simulink library "SimCoreLib"  (R2016b)
settings: Solver=VariableStepAuto  StartTime=0.0  StopTime=10.0  RelTol=1e-3
undefined symbols (not defined in the file or in its folder): Earth, Env, inertia, m, mass_0, s, Sim, WGS84
undefined symbols (not defined in the file): AC, TrimCondition
libraries: OpenFlightUtilLib x19, SimCoreLib x5, Navigation_Lib x5, aerolib6dofsys x4, aerolibconvert2 x2, SimCore_Lib x1, aerolibutil x1, simulink x1, aerolibtransform2 x1
settings Model: Creator=UAVLAB  LastModifiedBy=rega0051

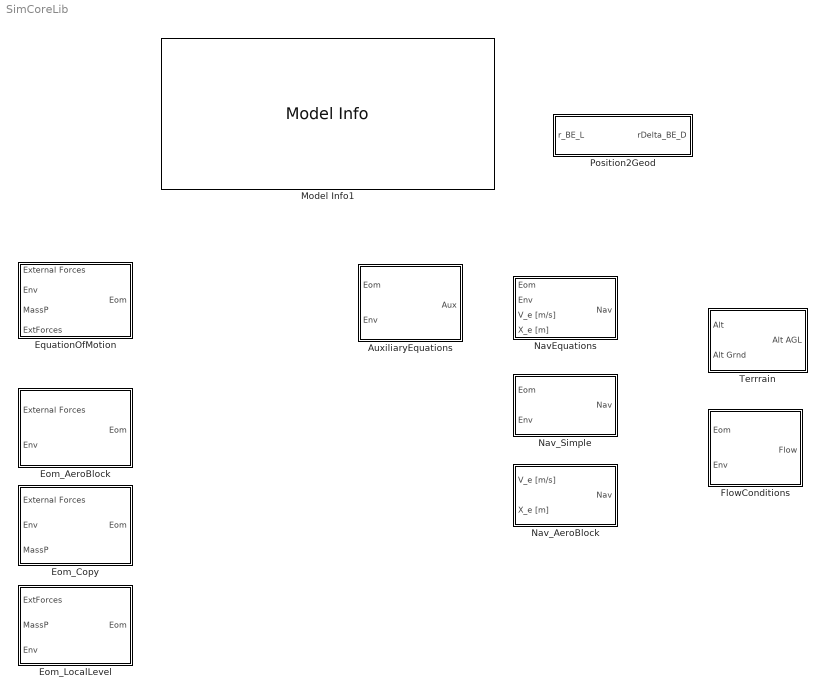
== system SimCoreLib ==
  AuxiliaryEquations : Subsystem
  Eom_AeroBlock : Subsystem  mask(6DoF EoM (Body Axis)){units=Metric (MKS), mtype=Fixed, rep=Euler Angles, xme_0=TrimCondition.InertialIni, Vm_0=TrimCondition.VelocitiesIni, eul_0=TrimCondition.AttitudeIni, pm_0=TrimCondition.RatesIni, mass_0=AC.MassP.mass_kg, mass_e=0.5, mass_f=2.0, inertia=AC.MassP.I_B_kgm2, inertia_e=eye(3), inertia_f=2*eye(3), k_quat=1.0}
      mask prompts: mtype "Mass type:"; rep "Representation:"; xme_0 "Initial position in inertial axes [Xe,Ye,Ze]:"; Vm_0 "Initial velocity in body axes [U,v,w]:"; eul_0 "Initial Euler orientation [roll, pitch, yaw]:"; pm_0 "Initial body rotation rates [p,q,r]:"; mass_0 "Initial mass:"; mass_e "Empty mass:"; mass_f "Full mass:"; inertia_e "Empty inertia matrix:"; inertia_f "Full inertia matrix:"; k_quat "Gain for quaternion normalization:"
      mask help:
      | Integrate the six-degrees-of-freedom equations of motion in body axis.
      |
      | This block has been modified from the original Aerospace Blockset
      | implementation. The inertial position vector (Xe) is no longer computed.
      | The original block did not have a way to add steady state winds to the
      | inertial velocities (Ve) prior to integrating to get Xe. Therefore, this
      | step is performed in the Auxiliary Equations block.
      mask Help: eval('asbhelp(''sixdof_euler_angles'')');
      mask TypeOptions units: Metric (MKS) | English (Velocity in ft/s) | English (Velocity in kts)
      mask TypeOptions mtype: Fixed | Simple Variable | Custom Variable
      mask Callback mtype: aeroicon('aeroblk6dofbody');
      mask TypeOptions rep: Euler Angles | Quaternion
      mask Callback rep: aeroicon('aeroblk6dofbody');
  Eom_Copy : Subsystem  mask{xme_0=TrimCondition.InertialIni, Vm_0=TrimCondition.VelocitiesIni, eul_0=TrimCondition.AttitudeIni, pm_0=TrimCondition.RatesIni, k_quat=1.0}
      mask prompts: xme_0 "Initial position in inertial axes [Xe,Ye,Ze]:"; Vm_0 "Initial velocity in body axes [U,v,w]:"; eul_0 "Initial Euler orientation [roll, pitch, yaw]:"; pm_0 "Initial body rotation rates [p,q,r]:"; k_quat "Gain for quaternion normalization:"
  Eom_LocalLevel : Subsystem
  EquationOfMotion : Subsystem  BlockChoice=Eom_AeroBlock
      settings: TemplateBlock=self  MemberBlocks=Eom_AeroBlock,Eom_Copy,Eom_LocalLevel
  FlowConditions : Subsystem
  Model Info1 : simulink/Model-Wide Utilities/Model Info  Frame=on  DisplayStringWithTags=|  HorizontalTextAlignment=Left  LeftAlignmentValue=0.02  SourceBlockDiagram=SimCoreLib  TagMaxNumber=20
      | MODEL INFORMATION
      | Simulation Core Library (%<ModelName>)
      | 
      | University of Minnesota
      | Aerospace Engineering and Mechanics
      | Copyright 2017 Regents of the University of Minnesota. All rights reserved.
      | 
      | == Update Info ==
      | Last modified by %<LastModifiedBy> on %<LastModificationDate>
  NavEquations : Subsystem  BlockChoice=Nav_Simple
      settings: TemplateBlock=self  MemberBlocks=Nav_AeroBlock,Nav_Simple
  Nav_AeroBlock : Subsystem
  Nav_Simple : Subsystem
  Position2Geod : Subsystem
  Terrrain : Subsystem

== system SimCoreLib/AuxiliaryEquations ==
  Eom : Inport  OutDataTypeStr=Bus: BusEom
  Env : Inport  Port=2  OutDataTypeStr=Bus: BusEnv
  Bus Creator2 : BusCreator  Inputs=2  OutDataTypeStr=Bus: BusAux
      settings: AttributesFormatString=%<OutDataTypeStr>  InheritFromInputs=off
  FlowConditions : SimCoreLib/FlowConditions
  Nav_Simple : SimCoreLib/Nav_Simple
  Aux : Outport
  wires:
  Bus Creator2/1 -> Aux/1  "BusAux"
  Env/1 -> FlowConditions/2, Nav_Simple/2
  Nav_Simple/1 -> Bus Creator2/2
  FlowConditions/1 -> Bus Creator2/1
  Eom/1 -> FlowConditions/1, Nav_Simple/1

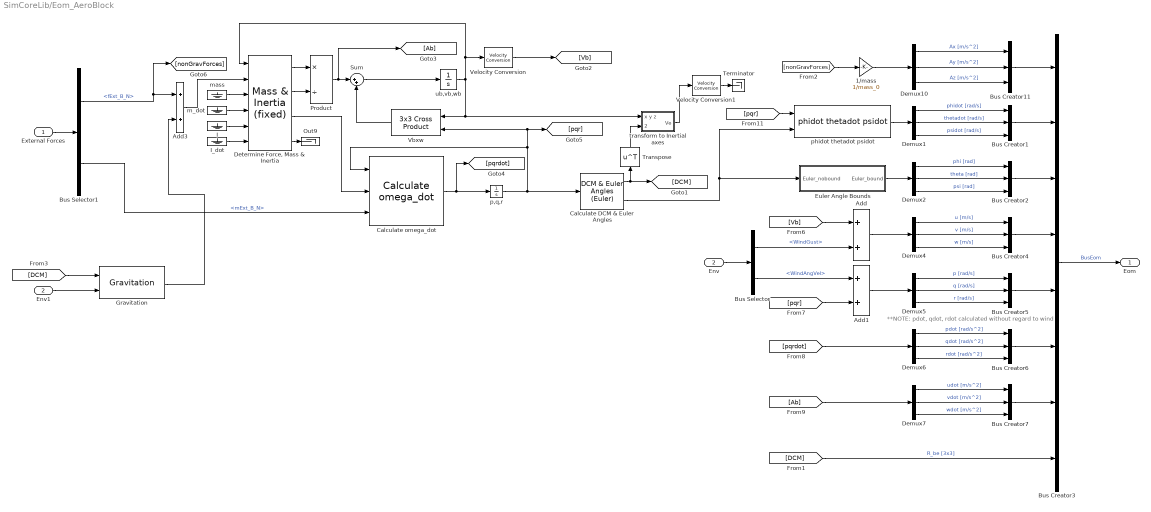
== system SimCoreLib/Eom_AeroBlock ==
  note: **NOTE: pdot, qdot, rdot calculated without regard to wind
  External Forces : Inport
  Env : Inport  Port=2
  1/mass : Gain  Gain=1/mass_0
  Add : Sum
  Add1 : Sum
  Add3 : Sum
  Bus Creator{1..2,4..7,11} (7 alike) : BusCreator  Inputs=3
  Bus Selector : BusSelector  OutputSignals=WindGust,WindAngVel
  Bus Selector1 : BusSelector  OutputSignals=fExt_B_N,mExt_B_N
  Bus Creator3 : BusCreator  Inputs=8  OutDataTypeStr=Bus: BusEom
      settings: AttributesFormatString=%<OutDataTypeStr>  InheritFromInputs=off
  Calculate DCM & Euler Angles : aerolib6dofsys/DCM & Euler Angles (Euler)  SystemSampleTime=-1
  Calculate omega_dot : aerolib6dofsys/Calculate omega_dot  SystemSampleTime=-1
  Demux{1..2,4..7,10} (7 alike) : Demux  Outputs=3
  "Determine Force, Mass & Inertia" : aerolib6dofsys/Mass & Inertia (fixed)  SystemSampleTime=-1
  Env1 : InportShadow  Port=2
  Euler Angle Bounds : Subsystem
  Gravitation : SimCore_Lib/Gravitation
  I : Ground
  I_dot : Ground
  Out9 : Terminator
  Product : Product  Inputs=*/  SaturateOnIntegerOverflow=on  OutDataTypeStr=Inherit: Same as first input
  Sum : Sum  Inputs=|++  SaturateOnIntegerOverflow=on
  Terminator : Terminator
  Transpose : Math  Operator=transpose  SaturateOnIntegerOverflow=on
  Vbxw : aerolibutil/3x3 Cross Product
  Velocity Conversion : aerolibconvert2/Velocity Conversion  IU=m/s  OU=m/s
  Velocity Conversion1 : aerolibconvert2/Velocity Conversion  IU=m/s  OU=m/s
  m_dot : Ground
  mass : Ground
  "p,q,r " : Integrator  InitialCondition=pm_0
  phidot thetadot psidot : aerolib6dofsys/DCM & Euler Angles (Euler)/phidot thetadot psidot
  "transform to Inertial axes " : Subsystem  mask(Vector Transformation){}
      mask Display: disp('L_EB')
  ub,vb,wb : Integrator  InitialCondition=convvel(Vm_0,'m/s','m/s')
  Eom : Outport
  wires:
  [DCM] -> Gravitation/1
  Env1/1 -> Gravitation/2
  Gravitation/1 -> Add3/2
  "Determine Force, Mass & Inertia"/1 -> Product/1
  I_dot/1 -> "Determine Force, Mass & Inertia"/6
  I/1 -> "Determine Force, Mass & Inertia"/5
  Calculate omega_dot/1 -> [pqrdot], "p,q,r "/1
  "Determine Force, Mass & Inertia"/4 -> Out9/1
  m_dot/1 -> "Determine Force, Mass & Inertia"/4
  "Determine Force, Mass & Inertia"/2 -> Product/2
  mass/1 -> "Determine Force, Mass & Inertia"/3
  Transpose/1 -> "transform to Inertial axes "/2(transform coefficients)
  Calculate DCM & Euler Angles/1 -> [DCM], Transpose/1
  Product/1 -> [Ab], Sum/1
  "p,q,r "/1 -> Calculate omega_dot/1, [pqr], Vbxw/2, Calculate DCM & Euler Angles/1
  "transform to Inertial axes "/1(Ve) -> Velocity Conversion1/1
  Sum/1 -> ub,vb,wb/1
  ub,vb,wb/1 -> "Determine Force, Mass & Inertia"/1, Velocity Conversion/1, Vbxw/1, "transform to Inertial axes "/1(x y z)
  Vbxw/1 -> Sum/2
  "Determine Force, Mass & Inertia"/3 -> Calculate omega_dot/2
  Velocity Conversion/1 -> [Vb]
  Velocity Conversion1/1 -> Terminator/1
  Env/1 -> Bus Selector/1
  Bus Selector/1 -> Add/2  "<WindGust>"
  Bus Selector/2 -> Add1/1  "<WindAngVel>"
  [Vb] -> Add/1
  Add/1 -> Demux4/1
  Demux4/3 -> Bus Creator4/3  "w [m/s]"
  Demux4/2 -> Bus Creator4/2  "v [m/s]"
  Demux4/1 -> Bus Creator4/1  "u [m/s]"
  [pqr] -> Add1/2
  Demux5/3 -> Bus Creator5/3  "r [rad/s]"
  Demux5/2 -> Bus Creator5/2  "q [rad/s]"
  Demux5/1 -> Bus Creator5/1  "p [rad/s]"
  Add1/1 -> Demux5/1
  [pqrdot] -> Demux6/1
  Demux6/3 -> Bus Creator6/3  "rdot [rad/s^2]"
  Demux6/2 -> Bus Creator6/2  "qdot [rad/s^2]"
  Demux6/1 -> Bus Creator6/1  "pdot [rad/s^2]"
  [Ab] -> Demux7/1
  Demux7/3 -> Bus Creator7/3  "wdot [m/s^2]"
  Demux7/2 -> Bus Creator7/2  "vdot [m/s^2]"
  Demux7/1 -> Bus Creator7/1  "udot [m/s^2]"
  Demux1/3 -> Bus Creator1/3  "psidot [rad/s]"
  Demux1/2 -> Bus Creator1/2  "thetadot [rad/s]"
  Demux1/1 -> Bus Creator1/1  "phidot [rad/s]"
  phidot thetadot psidot/1 -> Demux1/1
  [pqr] -> phidot thetadot psidot/1
  Calculate DCM & Euler Angles/2 -> Euler Angle Bounds/1(Euler_nobound), phidot thetadot psidot/2
  Demux2/3 -> Bus Creator2/3  "psi [rad]"
  Demux2/2 -> Bus Creator2/2  "theta [rad]"
  Demux2/1 -> Bus Creator2/1  "phi [rad]"
  Euler Angle Bounds/1(Euler_bound) -> Demux2/1
  [nonGravForces] -> 1/mass/1
  1/mass/1 -> Demux10/1
  Demux10/1 -> Bus Creator11/1  "Ax [m/s^2]"
  Demux10/2 -> Bus Creator11/2  "Ay [m/s^2]"
  Demux10/3 -> Bus Creator11/3  "Az [m/s^2]"
  External Forces/1 -> Bus Selector1/1
  Bus Selector1/1 -> [nonGravForces], Add3/1  "<fExt_B_N>"
  Add3/1 -> "Determine Force, Mass & Inertia"/2
  Bus Selector1/2 -> Calculate omega_dot/3  "<mExt_B_N>"
  Bus Creator3/1 -> Eom/1  "BusEom"
  Bus Creator4/1 -> Bus Creator3/4
  Bus Creator5/1 -> Bus Creator3/5
  Bus Creator6/1 -> Bus Creator3/6
  Bus Creator7/1 -> Bus Creator3/7
  Bus Creator1/1 -> Bus Creator3/2
  Bus Creator2/1 -> Bus Creator3/3
  Bus Creator11/1 -> Bus Creator3/1
  [DCM] -> Bus Creator3/8  "R_be [3x3]"

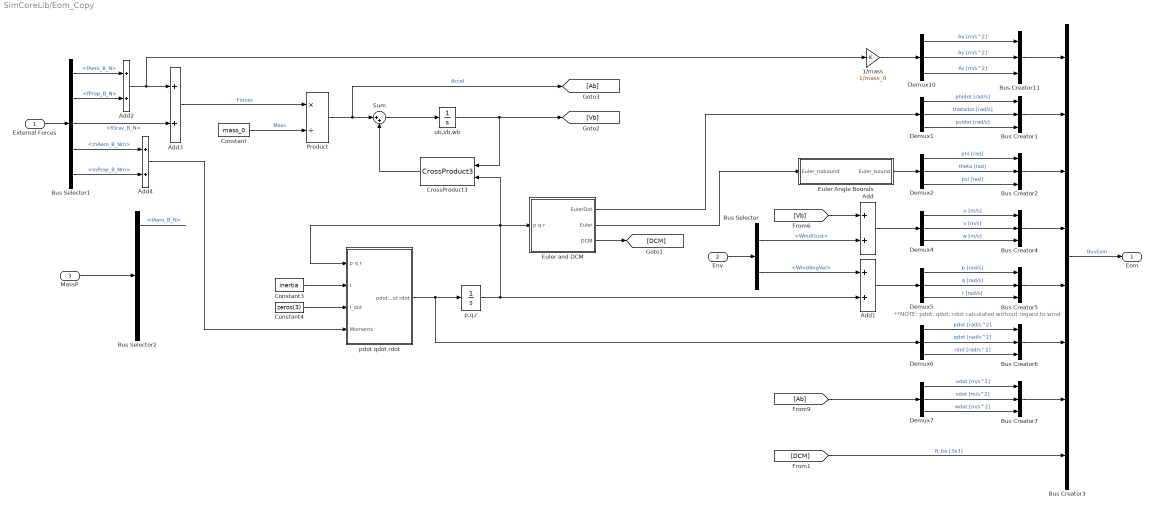
== system SimCoreLib/Eom_Copy ==
  note: **NOTE: pdot, qdot, rdot calculated without regard to wind
  External Forces : Inport
  Env : Inport  Port=2  OutDataTypeStr=Bus: EnvData
  MassP : Inport  Port=3
  1/mass : Gain  Gain=1/mass_0
  Add{,1..4} (5 alike) : Sum
  Bus Creator{1..2,4..7,11} (7 alike) : BusCreator  Inputs=3
  Bus Selector : BusSelector  OutputSignals=WindGust,WindAngVel
  Bus Selector1 : BusSelector  OutputSignals=fAero_B_N,fProp_B_N,fGrav_B_N,mAero_B_Nm,mProp_B_Nm
  Bus Selector2 : BusSelector  OutputSignals=fAero_B_N,fProp_B_N,fGrav_B_N,mAero_B_Nm,mProp_B_Nm
  Bus Creator3 : BusCreator  Inputs=8  OutDataTypeStr=Bus: BusEom
      settings: AttributesFormatString=%<OutDataTypeStr>  InheritFromInputs=off
  Constant : Constant  Value=mass_0  OutDataTypeStr=Inherit: Inherit via back propagation
  Constant3 : Constant  Value=inertia  OutDataTypeStr=Inherit: Inherit via back propagation
  Constant4 : Constant  Value=zeros(3)
  CrossProduct3 : OpenFlightUtilLib/Math/CrossProduct3
  Demux{1..2,4..7,10} (7 alike) : Demux  Outputs=3
  Euler Angle Bounds : Subsystem
  Euler and DCM : Subsystem
  Product : Product  Inputs=*/  SaturateOnIntegerOverflow=on  OutDataTypeStr=Inherit: Same as first input
  Sum : Sum  Inputs=|++  SaturateOnIntegerOverflow=on
  "p,q,r " : Integrator  InitialCondition=pm_0
  pdot qdot rdot : Subsystem
  ub,vb,wb : Integrator  InitialCondition=Vm_0
  Eom : Outport  OutDataTypeStr=Bus: RigidStates
  wires:
  Constant3/1 -> pdot qdot rdot/2(I)
  Constant4/1 -> pdot qdot rdot/3(I_dot)
  ub,vb,wb/1 -> CrossProduct3/1, [Vb]
  Add3/1 -> Product/1  "Forces"
  Constant/1 -> Product/2  "Mass"
  Euler and DCM/3(DCM) -> [DCM]
  Product/1 -> Sum/1, [Ab]  "Accel"
  Sum/1 -> ub,vb,wb/1
  CrossProduct3/1 -> Sum/2
  Env/1 -> Bus Selector/1
  Bus Selector/1 -> Add/2  "<WindGust>"
  Bus Selector/2 -> Add1/1  "<WindAngVel>"
  [Vb] -> Add/1
  Add/1 -> Demux4/1
  Demux4/3 -> Bus Creator4/3  "w [m/s]"
  Demux4/2 -> Bus Creator4/2  "v [m/s]"
  Demux4/1 -> Bus Creator4/1  "u [m/s]"
  "p,q,r "/1 -> pdot qdot rdot/1(p q r), CrossProduct3/2, Euler and DCM/1("p q r "), Add1/2
  Demux5/3 -> Bus Creator5/3  "r [rad/s]"
  Demux5/2 -> Bus Creator5/2  "q [rad/s]"
  Demux5/1 -> Bus Creator5/1  "p [rad/s]"
  Add1/1 -> Demux5/1
  pdot qdot rdot/1(pdot qdot rdot) -> Demux6/1, "p,q,r "/1
  Demux6/3 -> Bus Creator6/3  "rdot [rad/s^2]"
  Demux6/2 -> Bus Creator6/2  "qdot [rad/s^2]"
  Demux6/1 -> Bus Creator6/1  "pdot [rad/s^2]"
  [Ab] -> Demux7/1
  Demux7/3 -> Bus Creator7/3  "wdot [m/s^2]"
  Demux7/2 -> Bus Creator7/2  "vdot [m/s^2]"
  Demux7/1 -> Bus Creator7/1  "udot [m/s^2]"
  Demux1/3 -> Bus Creator1/3  "psidot [rad/s]"
  Demux1/2 -> Bus Creator1/2  "thetadot [rad/s]"
  Demux1/1 -> Bus Creator1/1  "phidot [rad/s]"
  Euler and DCM/1(EulerDot) -> Demux1/1
  Euler and DCM/2(Euler) -> Euler Angle Bounds/1(Euler_nobound)
  Demux2/3 -> Bus Creator2/3  "psi [rad]"
  Demux2/2 -> Bus Creator2/2  "theta [rad]"
  Demux2/1 -> Bus Creator2/1  "phi [rad]"
  Euler Angle Bounds/1(Euler_bound) -> Demux2/1
  Add2/1 -> Add3/1, 1/mass/1
  1/mass/1 -> Demux10/1
  Demux10/1 -> Bus Creator11/1  "Ax [m/s^2]"
  Demux10/2 -> Bus Creator11/2  "Ay [m/s^2]"
  Demux10/3 -> Bus Creator11/3  "Az [m/s^2]"
  External Forces/1 -> Bus Selector1/1
  Bus Selector1/1 -> Add2/1  "<fAero_B_N>"
  Bus Selector1/2 -> Add2/2  "<fProp_B_N>"
  Bus Selector1/3 -> Add3/2  "<fGrav_B_N>"
  Bus Selector1/4 -> Add4/1  "<mAero_B_Nm>"
  Bus Selector1/5 -> Add4/2  "<mProp_B_Nm>"
  Add4/1 -> pdot qdot rdot/4(Moments)
  Bus Creator3/1 -> Eom/1  "BusEom"
  Bus Creator4/1 -> Bus Creator3/4
  Bus Creator5/1 -> Bus Creator3/5
  Bus Creator6/1 -> Bus Creator3/6
  Bus Creator7/1 -> Bus Creator3/7
  Bus Creator1/1 -> Bus Creator3/2
  Bus Creator2/1 -> Bus Creator3/3
  Bus Creator11/1 -> Bus Creator3/1
  [DCM] -> Bus Creator3/8  "R_be [3x3]"
  MassP/1 -> Bus Selector2/1
  Bus Selector2/1 -> ?  "<fAero_B_N>"

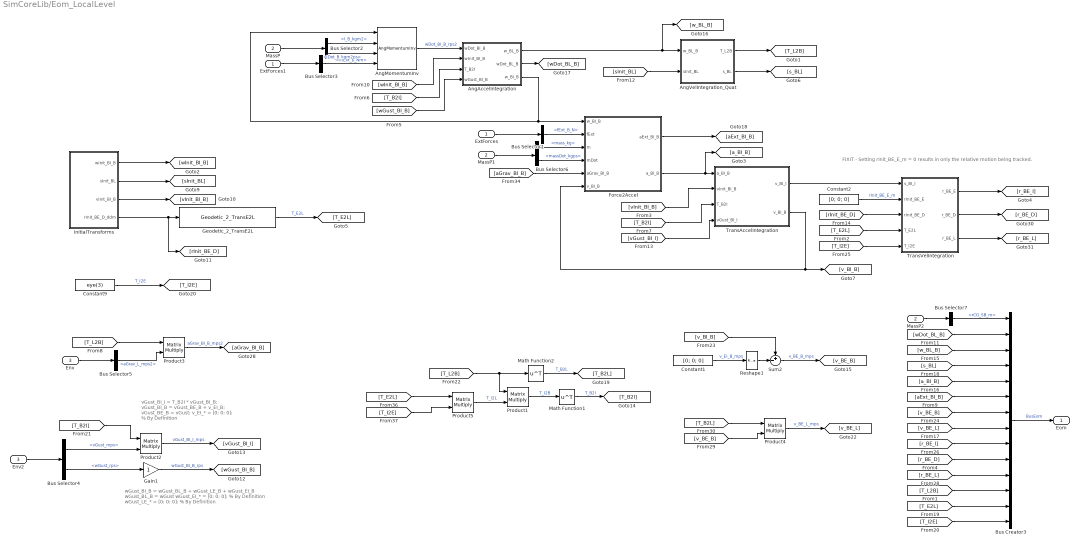
== system SimCoreLib/Eom_LocalLevel ==
  note: wGust_BI_B = wGust_BL_B + wGust_LE_B + wGust_EI_B
      | wGust_BL_B = wGust
      | wGust_EI_* = [0; 0; 0]; % By Definition
      | wGust_LE_* = [0; 0; 0]; % By Definition
  note: vGust_BI_I = T_B2I * vGust_BI_B;
      | vGust_BI_B = vGust_BE_B + v_EI_B;
      | vGust_BE_B = vGust;
      | v_EI_* = [0; 0; 0]; % By Definition
  note: FIXIT - Setting rInit_BE_E_m = 0 results in only the relative motion being tracked.
  ExtForces : Inport
  MassP : Inport  Port=2
  Env : Inport  Port=3  OutDataTypeStr=Bus: BusEnv
  AngAccelIntegration : Subsystem
  AngMomentumInv : OpenFlightUtilLib/Kinematics and Dynamics/AngMomentumInv
  AngVelIntegration_Quat : Subsystem
  Bus Selector1 : BusSelector  OutputSignals=fExt_B_N
  Bus Selector2 : BusSelector  OutputSignals=I_B_kgm2,IDot_B_kgm2ps
  Bus Selector3 : BusSelector  OutputSignals=mExt_B_Nm
  Bus Selector4 : BusSelector  OutputSignals=BusAtmos.vGust_mps,BusAtmos.wGust_rps
  Bus Selector5 : BusSelector  OutputSignals=BusGrav.aGrav_L_mps2
  Bus Selector6 : BusSelector  OutputSignals=mass_kg,massDot_kgps
  Bus Selector7 : BusSelector  OutputSignals=rCG_SB_m
  Bus Creator3 : BusCreator  Inputs=14  OutDataTypeStr=Bus: BusEom
      settings: AttributesFormatString=%<OutDataTypeStr>
  Constant1 : Constant  Value=[0; 0; 0]
      settings: AttributesFormatString=%<Value>
  Constant2 : Constant  Value=[0; 0; 0]
      settings: AttributesFormatString=%<Value>
  Constant9 : Constant  Value=eye(3)
      settings: AttributesFormatString=%<Value>
  Env2 : InportShadow  Port=3  OutDataTypeStr=Bus: BusEnv
  ExtForces1 : InportShadow
  Force2Accel : Subsystem
  Gain1 : Gain
  Geodetic_2_TransE2L : OpenFlightUtilLib/Transformations/Geodetic_2_TransE2L
  InitialTransforms : Subsystem
  MassP1 : InportShadow  Port=2
  MassP2 : InportShadow  Port=2
  Math Function1 : Math  Operator=transpose  SaturateOnIntegerOverflow=on
  Math Function2 : Math  Operator=transpose  SaturateOnIntegerOverflow=on
  Product{1..5} (5 alike) : Product  Inputs=**  Multiplication=Matrix(*)  RndMeth=Zero
  Reshape1 : Reshape  OutputDimensionality=Column vector (2-D)  OutputDimensions=[3,1]
  Sum2 : Sum  Inputs=+-|
  TransAccelIntegration : Subsystem
  TransVelIntegration : Subsystem
  Eom : Outport
  wires:
  Reshape1/1 -> Sum2/2
  Math Function2/1 -> [T_B2L]  "T_B2L"
  [v_BI_B] -> Sum2/1
  Constant1/1 -> Reshape1/1  "v_EI_B_mps"
  Sum2/1 -> [v_BE_B]  "v_BE_B_mps"
  [T_E2L] -> TransVelIntegration/4(T_E2L)
  Constant2/1 -> TransVelIntegration/2(rInit_BE_E)  "rInit_BE_E_m"
  [T_I2E] -> TransVelIntegration/5(T_I2E)
  [r_BE_I] -> Bus Creator3/9
  [v_BE_B] -> Bus Creator3/7
  [vGust_BI_I] -> TransAccelIntegration/4(vGust_BI_I)
  Gain1/1 -> [wGust_BI_B]  "wGust_BI_B_rps"
  Product2/1 -> [vGust_BI_I]  "vGust_BI_I_mps"
  [T_B2I] -> Product2/1
  Bus Selector4/2 -> Gain1/1  "<wGust_rps>"
  Env2/1 -> Bus Selector4/1
  [wGust_BI_B] -> AngAccelIntegration/4(wGust_BI_B)
  Bus Selector7/1 -> Bus Creator3/1  "<rCG_SB_m>"
  MassP2/1 -> Bus Selector7/1
  [T_E2L] -> Product5/1
  [T_I2E] -> Product5/2
  [rInit_BE_D] -> TransVelIntegration/3(rInit_BE_D)
  TransVelIntegration/3(r_BE_L) -> [r_BE_L]
  TransVelIntegration/2(r_BE_D) -> [r_BE_D]
  AngAccelIntegration/2(wDot_BL_B) -> [wDot_BL_B]
  [aGrav_BI_B] -> Force2Accel/5(aGrav_BI_B)
  Bus Selector4/1 -> Product2/2  "<vGust_mps>"
  Product5/1 -> Product1/2  "T_I2L"
  [T_B2L] -> Product4/1
  [v_BE_B] -> Product4/2
  [r_BE_L] -> Bus Creator3/11
  Product4/1 -> [v_BE_L]  "v_BE_L_mps"
  [T_L2B] -> Product1/1, Math Function2/1
  Constant9/1 -> [T_I2E]  "T_I2E"
  Geodetic_2_TransE2L/1 -> [T_E2L]  "T_E2L"
  Force2Accel/1(aExt_BI_B) -> [aExt_BI_B]
  [T_I2E] -> Bus Creator3/14
  [T_E2L] -> Bus Creator3/13
  AngAccelIntegration/1(w_BL_B) -> AngVelIntegration_Quat/1(w_BL_B), [w_BL_B]
  [v_BE_L] -> Bus Creator3/8
  [aExt_BI_B] -> Bus Creator3/6
  [wDot_BL_B] -> Bus Creator3/2
  [w_BL_B] -> Bus Creator3/3
  [r_BE_D] -> Bus Creator3/10
  [a_BI_B] -> Bus Creator3/5
  [s_BL] -> Bus Creator3/4
  MassP1/1 -> Bus Selector6/1
  [wInit_BI_B] -> AngAccelIntegration/2(wInit_BI_B)
  Bus Selector3/1 -> AngMomentumInv/4  "<mExt_B_Nm>"
  Bus Selector2/2 -> AngMomentumInv/3  "<IDot_B_kgm2ps>"
  Bus Selector2/1 -> AngMomentumInv/2  "<I_B_kgm2>"
  AngMomentumInv/1 -> AngAccelIntegration/1(wDot_BI_B)  "wDot_BI_B_rps2"
  [vInit_BI_B] -> TransAccelIntegration/2(vInit_BI_B)
  TransAccelIntegration/2(v_BI_B) -> Force2Accel/6(v_BI_B), [v_BI_B]
  Force2Accel/2(a_BI_B) -> TransAccelIntegration/1(a_BI_B), [a_BI_B]
  AngVelIntegration_Quat/2(s_BL) -> [s_BL]
  [sInit_BL] -> AngVelIntegration_Quat/2(sInit_BL)
  [T_L2B] -> Product3/1
  Bus Selector5/1 -> Product3/2  "<aGrav_L_mps2>"
  Env/1 -> Bus Selector5/1
  ExtForces1/1 -> Bus Selector3/1
  MassP/1 -> Bus Selector2/1
  [T_L2B] -> Bus Creator3/12
  Bus Creator3/1 -> Eom/1  "BusEom"
  Bus Selector1/1 -> Force2Accel/2(fExt)  "<fExt_B_N>"
  ExtForces/1 -> Bus Selector1/1
  AngVelIntegration_Quat/1(T_L2B) -> [T_L2B]
  Product3/1 -> [aGrav_BI_B]  "aGrav_BI_B_mps2"
  Bus Selector6/1 -> Force2Accel/3(m)  "<mass_kg>"
  Bus Selector6/2 -> Force2Accel/4(mDot)  "<massDot_kgps>"
  AngAccelIntegration/3(w_BI_B) -> AngMomentumInv/1, Force2Accel/1(w_BI_B)
  TransAccelIntegration/1(v_BI_I) -> TransVelIntegration/1(v_BI_I)
  TransVelIntegration/1(r_BE_E) -> [r_BE_I]
  [T_B2I] -> AngAccelIntegration/3(T_B2I)
  [T_B2I] -> TransAccelIntegration/3(T_B2I)
  Product1/1 -> Math Function1/1  "T_I2B"
  Math Function1/1 -> [T_B2I]  "T_B2I"
  InitialTransforms/1(wInit_BI_B) -> [wInit_BI_B]
  InitialTransforms/2(sInit_BL) -> [sInit_BL]
  InitialTransforms/3(vInit_BI_B) -> [vInit_BI_B]
  InitialTransforms/4(rInit_BE_D_ddm) -> Geodetic_2_TransE2L/1, [rInit_BE_D]

== system SimCoreLib/EquationOfMotion ==
  External Forces : Inport
  Env : Inport  Port=2
  MassP : Inport  Port=3
  ExtForces : Inport  Port=4
  Eom_AeroBlock : SimCoreLib/Eom_AeroBlock  units=Metric (MKS)  mtype=Fixed  rep=Euler Angles  xme_0=TrimCondition.InertialIni  Vm_0=TrimCondition.VelocitiesIni  eul_0=TrimCondition.AttitudeIni  pm_0=TrimCondition.RatesIni  mass_0=AC.MassP.mass_kg  mass_e=0.5  mass_f=2.0  inertia=AC.MassP.I_B_kgm2  inertia_e=eye(3)  inertia_f=2*eye(3)  k_quat=1.0
  term3 : Terminator
  term4 : Terminator
  Eom : Outport
  wires:
  External Forces/1 -> Eom_AeroBlock/1
  Env/1 -> Eom_AeroBlock/2
  Eom_AeroBlock/1 -> Eom/1
  MassP/1 -> term3/1
  ExtForces/1 -> term4/1

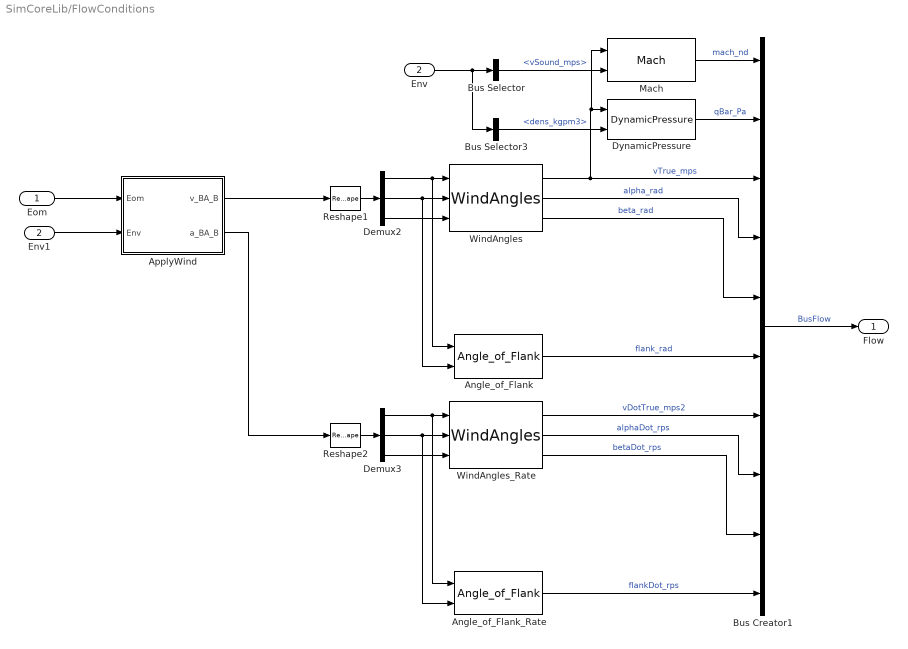
== system SimCoreLib/FlowConditions ==
  Eom : Inport
  Env : Inport  Port=2
  Angle_of_Flank : OpenFlightUtilLib/Air Data/Angle_of_Flank
  Angle_of_Flank_Rate : OpenFlightUtilLib/Air Data/Angle_of_Flank
  ApplyWind : Subsystem
  Bus Creator1 : BusCreator  Inputs=10  OutDataTypeStr=Bus: BusFlow
      settings: InheritFromInputs=off
  Bus Selector : BusSelector  OutputSignals=BusAtmos.vSound_mps
  Bus Selector3 : BusSelector  OutputSignals=BusAtmos.dens_kgpm3
  Demux2 : Demux  Outputs=3
  Demux3 : Demux  Outputs=3
  DynamicPressure : OpenFlightUtilLib/Air Data/DynamicPressure
  Env1 : InportShadow  Port=2
  Mach : OpenFlightUtilLib/Air Data/Mach
  Reshape1 : Reshape  OutputDimensions=[3,1]
  Reshape2 : Reshape  OutputDimensions=[3,1]
  WindAngles : OpenFlightUtilLib/Air Data/WindAngles
  WindAngles_Rate : OpenFlightUtilLib/Air Data/WindAngles
  Flow : Outport
  wires:
  Reshape2/1 -> Demux3/1
  Reshape1/1 -> Demux2/1
  ApplyWind/2(a_BA_B) -> Reshape2/1
  Env1/1 -> ApplyWind/2(Env)
  Eom/1 -> ApplyWind/1(Eom)
  WindAngles_Rate/2 -> Bus Creator1/8  "alphaDot_rps"
  Demux3/2 -> Angle_of_Flank_Rate/2, WindAngles_Rate/2
  WindAngles_Rate/1 -> Bus Creator1/7  "vDotTrue_mps2"
  Demux3/3 -> WindAngles_Rate/3
  Demux3/1 -> Angle_of_Flank_Rate/1, WindAngles_Rate/1
  WindAngles_Rate/3 -> Bus Creator1/9  "betaDot_rps"
  WindAngles/3 -> Bus Creator1/5  "beta_rad"
  Angle_of_Flank/1 -> Bus Creator1/6  "flank_rad"
  Angle_of_Flank_Rate/1 -> Bus Creator1/10  "flankDot_rps"
  Bus Creator1/1 -> Flow/1  "BusFlow"
  WindAngles/2 -> Bus Creator1/4  "alpha_rad"
  Demux2/2 -> Angle_of_Flank/2, WindAngles/2
  Demux2/1 -> Angle_of_Flank/1, WindAngles/1
  WindAngles/1 -> Mach/1, DynamicPressure/1, Bus Creator1/3  "vTrue_mps"
  Demux2/3 -> WindAngles/3
  DynamicPressure/1 -> Bus Creator1/2  "qBar_Pa"
  Bus Selector3/1 -> DynamicPressure/2  "<dens_kgpm3>"
  Env/1 -> Bus Selector3/1, Bus Selector/1
  Bus Selector/1 -> Mach/2  "<vSound_mps>"
  Mach/1 -> Bus Creator1/1  "mach_nd"
  ApplyWind/1(v_BA_B) -> Reshape1/1

== system SimCoreLib/NavEquations ==
  Eom : Inport
  Env : Inport  Port=2
  V_e [m/s] : Inport  Port=3
  X_e [m] : Inport  Port=4
  Nav_Simple : SimCoreLib/Nav_Simple
  term3 : Terminator
  term4 : Terminator
  Nav : Outport
  wires:
  Eom/1 -> Nav_Simple/1
  Env/1 -> Nav_Simple/2
  Nav_Simple/1 -> Nav/1
  V_e [m/s]/1 -> term3/1
  X_e [m]/1 -> term4/1

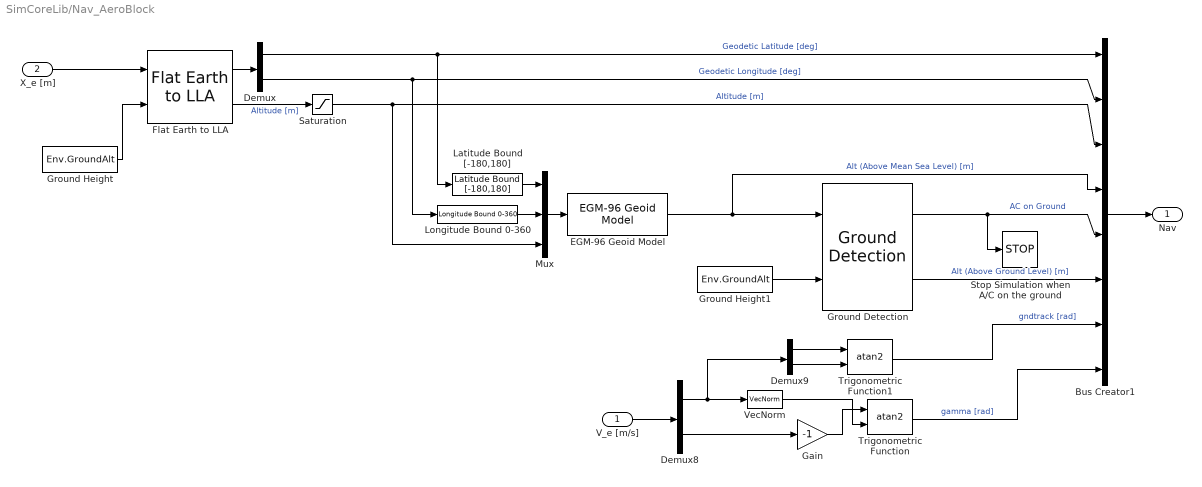
== system SimCoreLib/Nav_AeroBlock ==
  V_e [m/s] : Inport
  X_e [m] : Inport  Port=2
  Bus Creator1 : BusCreator  Inputs=8  OutDataTypeStr=Bus: Nav
      settings: InheritFromInputs=off
  Demux : Demux  Outputs=2
  Demux8 : Demux  Outputs=[2 1]
  Demux9 : Demux  Outputs=2
  EGM-96 Geoid Model : Navigation_Lib/Navigation/EGM-96 Geoid Model
  Flat Earth to LLA : aerolibtransform2/Flat Earth to LLA  units=Metric (MKS)  ptype=Earth (WGS84)  F=1/298.257223563  R=6378137  LL0=TrimCondition.LLIni  psi=0
  Gain : Gain  Gain=-1
  Ground Detection : Navigation_Lib/Navigation/Ground Detection
  Ground Height : Constant  Value=Env.GroundAlt
  Ground Height1 : Constant  Value=Env.GroundAlt
  Latitude Bound [-180,180] : Navigation_Lib/Navigation/Latitude Bound [-180,180]
  Longitude Bound 0-360 : Navigation_Lib/Navigation/Longitude Bound 0-360
  Mux : Mux  Inputs=3
  Saturation : Saturate  UpperLimit=Inf  LowerLimit=0
  Stop Simulation when A/C on the ground : Stop
  Trigonometric Function : Trigonometry  Operator=atan2
  Trigonometric Function1 : Trigonometry  Operator=atan2
  VecNorm : Navigation_Lib/Navigation/VecNorm
  Nav : Outport  OutDataTypeStr=Bus: Nav
  wires:
  Flat Earth to LLA/1 -> Demux/1
  Flat Earth to LLA/2 -> Saturation/1  "Altitude [m]"
  Demux/1 -> Bus Creator1/1, Latitude Bound [-180,180]/1  "Geodetic Latitude [deg]"
  Demux/2 -> Bus Creator1/2, Longitude Bound 0-360/1  "Geodetic Longitude [deg]"
  X_e [m]/1 -> Flat Earth to LLA/1
  Ground Height/1 -> Flat Earth to LLA/2
  Bus Creator1/1 -> Nav/1
  EGM-96 Geoid Model/1 -> Ground Detection/1, Bus Creator1/4  "Alt (Above Mean Sea Level) [m]"
  Ground Height1/1 -> Ground Detection/2
  Ground Detection/1 -> Stop Simulation when A/C on the ground/1, Bus Creator1/5  "AC on Ground"
  Saturation/1 -> Bus Creator1/3, Mux/3  "Altitude [m]"
  Mux/1 -> EGM-96 Geoid Model/1
  Ground Detection/2 -> Bus Creator1/6  "Alt (Above Ground Level) [m]"
  V_e [m/s]/1 -> Demux8/1
  Demux8/2 -> Gain/1
  VecNorm/1 -> Trigonometric Function/2
  Trigonometric Function/1 -> Bus Creator1/8  "gamma [rad]"
  Demux9/2 -> Trigonometric Function1/2
  Trigonometric Function1/1 -> Bus Creator1/7  "gndtrack [rad]"
  Demux8/1 -> VecNorm/1, Demux9/1
  Demux9/1 -> Trigonometric Function1/1
  Longitude Bound 0-360/1 -> Mux/2
  Latitude Bound [-180,180]/1 -> Mux/1
  Gain/1 -> Trigonometric Function/1

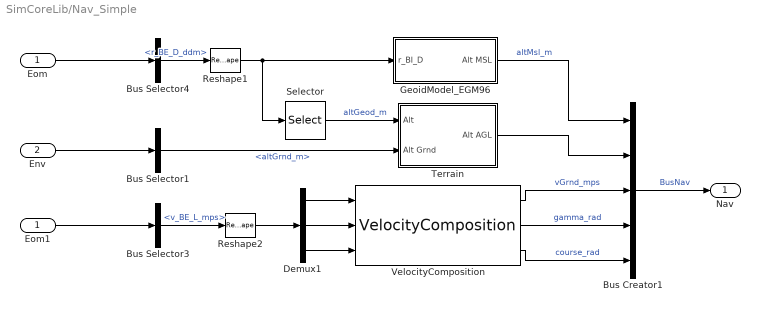
== system SimCoreLib/Nav_Simple ==
  Eom : Inport
  Env : Inport  Port=2
  Bus Creator1 : BusCreator  Inputs=5  OutDataTypeStr=Bus: BusNav
      settings: AttributesFormatString=%<OutDataTypeStr>  InheritFromInputs=off
  Bus Selector1 : BusSelector  OutputSignals=BusTerr.altGrnd_m
  Bus Selector3 : BusSelector  OutputSignals=v_BE_L_mps
  Bus Selector4 : BusSelector  OutputSignals=r_BE_D_ddm
  Demux1 : Demux  Outputs=3
  Eom1 : InportShadow
  GeoidModel_EGM96 : Subsystem  mask(EGM-96 geoid undulation model){}
      mask help: Computes the MSL (mean sea level) altitude as a function of position.
      mask init:
      | load('egm96');
      mask Help:
      | The block computes the mean-sea-level altitude relative to the WGS-84 geoid.
      | <P><B>Inputs:</B>
      | <LI>Position = the 3x1 vector of aircraft location [Latitude Longitude Altitude], in [rad rad m]</LI>
      | </P>
      | <P><B>Output:</B>
      | <LI>MSLAlt = the mean-sea-level altitude, in m</LI>
      | </P>
  Reshape1 : Reshape  OutputDimensions=[3,1]
  Reshape2 : Reshape  OutputDimensions=[3,1]
  Selector : Selector  InputPortWidth=3  IndexOptions=Index vector (dialog)  Indices=3  OutputSizes=1
  Terrain : Subsystem
  VelocityComposition : OpenFlightUtilLib/Transformations/VelocityComposition
  Nav : Outport
  wires:
  Reshape2/1 -> Demux1/1
  Reshape1/1 -> Selector/1, GeoidModel_EGM96/1(r_BI_D)
  Bus Selector4/1 -> Reshape1/1  "<r_BE_D_ddm>"
  Bus Selector3/1 -> Reshape2/1  "<v_BE_L_mps>"
  Eom1/1 -> Bus Selector3/1
  Bus Creator1/1 -> Nav/1  "BusNav"
  GeoidModel_EGM96/1(Alt MSL) -> Bus Creator1/1  "altMsl_m"
  Selector/1 -> Terrain/1(Alt)  "altGeod_m"
  Demux1/1 -> VelocityComposition/1
  Demux1/2 -> VelocityComposition/2
  Demux1/3 -> VelocityComposition/3
  VelocityComposition/1 -> Bus Creator1/3  "vGrnd_mps"
  VelocityComposition/2 -> Bus Creator1/4  "gamma_rad"
  VelocityComposition/3 -> Bus Creator1/5  "course_rad"
  Eom/1 -> Bus Selector4/1
  Terrain/1(Alt AGL) -> Bus Creator1/2
  Bus Selector1/1 -> Terrain/2(Alt Grnd)  "<altGrnd_m>"
  Env/1 -> Bus Selector1/1

== system SimCoreLib/Position2Geod ==
  r_BE_L : Inport
  Constant1 : Constant  Value=Env.Earth.radiusEquator_m
      settings: AttributesFormatString=%<Value>
  Constant2 : Constant  Value=Env.Earth.radiusPolar_m
      settings: AttributesFormatString=%<Value>
  Demux1 : Demux  Outputs=3
  Gain : Gain  Gain=180/pi
      settings: AttributesFormatString=%<Gain>
  Gain1 : Gain  Gain=-1
      settings: AttributesFormatString=%<Gain>
  Gain2 : Gain  Gain=180/pi
      settings: AttributesFormatString=%<Gain>
  Mux : Mux  Inputs=3
  Product : Product  Inputs=*/
  Product1 : Product  Inputs=*/
  rDelta_BE_D : Outport
  wires:
  Gain1/1 -> Mux/3
  Mux/1 -> rDelta_BE_D/1  "rDelta_BE_D_ddm"
  Demux1/3 -> Gain1/1
  Demux1/1 -> Product/1
  Constant2/1 -> Product/2
  r_BE_L/1 -> Demux1/1
  Gain2/1 -> Mux/1
  Product/1 -> Gain2/1
  Constant1/1 -> Product1/2
  Demux1/2 -> Product1/1
  Product1/1 -> Gain/1
  Gain/1 -> Mux/2

== system SimCoreLib/Terrrain ==
  Alt : Inport
  Alt Grnd : Inport  Port=2
  Sum : Sum  Inputs=|+-  SaturateOnIntegerOverflow=on  InputSameDT=on  OutDataTypeStr=Inherit: Same as first input
  Alt AGL : Outport
  wires:
  Alt/1 -> Sum/1
  Sum/1 -> Alt AGL/1  "altAgl_m"
  Alt Grnd/1 -> Sum/2

== system SimCoreLib/Eom_AeroBlock/Euler Angle Bounds ==
  Euler_nobound : Inport
  2pi Bound : Subsystem
  Demux : Demux  Outputs=3
  Mux : Mux  Inputs=3
  pi Bound : Subsystem
  pi/2 Bound : Subsystem
  Euler_bound : Outport
  wires:
  pi Bound/1(Out) -> Mux/2
  pi/2 Bound/1(Out) -> Mux/1
  Mux/1 -> Euler_bound/1
  Euler_nobound/1 -> Demux/1
  Demux/1 -> pi/2 Bound/1(In)
  Demux/2 -> pi Bound/1(In)
  Demux/3 -> 2pi Bound/1(In)
  2pi Bound/1(Out) -> Mux/3

== system SimCoreLib/Eom_AeroBlock/transform to Inertial axes  ==
  x y z : Inport
  transform coefficients : Inport  Port=2
  Product : Product  Multiplication=Matrix(*)  SaturateOnIntegerOverflow=on  InputSameDT=on  OutDataTypeStr=Inherit: Same as first input
  Reshape1 : Reshape  OutputDimensionality=Column vector (2-D)
  Reshape2 : Reshape
  Ve : Outport
  wires:
  Reshape2/1 -> Ve/1
  Reshape1/1 -> Product/2
  x y z/1 -> Reshape1/1
  transform coefficients/1 -> Product/1
  Product/1 -> Reshape2/1

== system SimCoreLib/Eom_Copy/Euler Angle Bounds ==
  Euler_nobound : Inport
  2pi Bound : Subsystem
  Demux : Demux  Outputs=3
  Mux : Mux  Inputs=3
  pi Bound : Subsystem
  pi/2 Bound : Subsystem
  Euler_bound : Outport
  wires:
  2pi Bound/1(Out) -> Mux/3
  Demux/3 -> 2pi Bound/1(In)
  Demux/2 -> pi Bound/1(In)
  Demux/1 -> pi/2 Bound/1(In)
  Euler_nobound/1 -> Demux/1
  Mux/1 -> Euler_bound/1
  pi/2 Bound/1(Out) -> Mux/1
  pi Bound/1(Out) -> Mux/2

== system SimCoreLib/Eom_Copy/Euler and DCM ==
  "p q r " : Inport
  DCM_321 : OpenFlightUtilLib/Transformations/DCM_321
  Demux3 : Demux  Outputs=3
  phi theta psi : Integrator  InitialCondition=eul_0
  phidot thetadot psidot : Subsystem
  EulerDot : Outport
  Euler : Outport  Port=2
  DCM : Outport  Port=3
  wires:
  Demux3/1 -> DCM_321/1
  Demux3/2 -> DCM_321/2
  Demux3/3 -> DCM_321/3
  DCM_321/1 -> DCM/1
  "p q r "/1 -> phidot thetadot psidot/2(p q r)
  phidot thetadot psidot/1(phidt thetadt psidt) -> phi theta psi/1, EulerDot/1
  phi theta psi/1 -> Euler/1, Demux3/1, phidot thetadot psidot/1(phi theta psi)

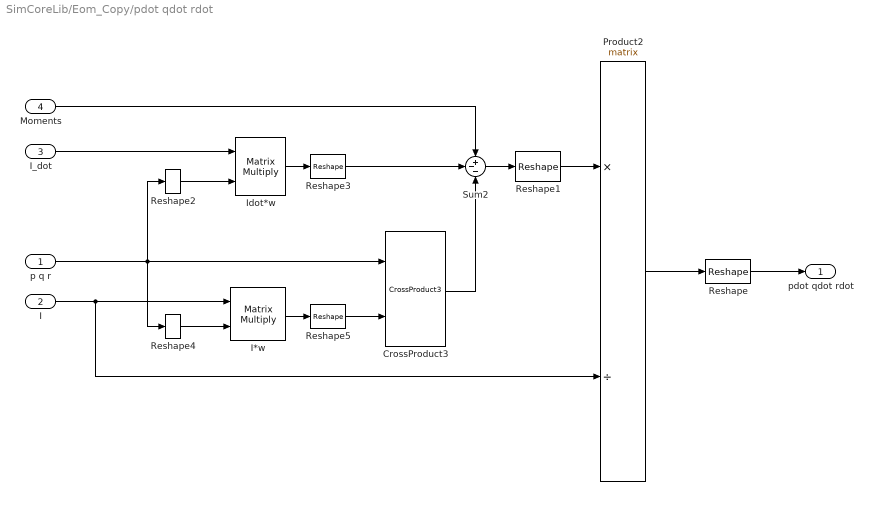
== system SimCoreLib/Eom_Copy/pdot qdot rdot ==
  p q r : Inport
  I : Inport  Port=2
  I_dot : Inport  Port=3
  Moments : Inport  Port=4
  CrossProduct3 : OpenFlightUtilLib/Math/CrossProduct3
  I*w : Product  Multiplication=Matrix(*)  SaturateOnIntegerOverflow=on  InputSameDT=on  OutDataTypeStr=Inherit: Same as first input
  Idot*w : Product  Multiplication=Matrix(*)  SaturateOnIntegerOverflow=on  InputSameDT=on  OutDataTypeStr=Inherit: Same as first input
  Product2 : Product  Inputs=*/  Multiplication=Matrix(*)  SaturateOnIntegerOverflow=on  OutDataTypeStr=Inherit: Same as first input
  Reshape : Reshape
  Reshape1 : Reshape  OutputDimensionality=Row vector (2-D)
  Reshape2 : Reshape  OutputDimensionality=Column vector (2-D)
  Reshape3 : Reshape
  Reshape4 : Reshape  OutputDimensionality=Column vector (2-D)
  Reshape5 : Reshape
  Sum2 : Sum  Inputs=+--  SaturateOnIntegerOverflow=on
  pdot qdot rdot : Outport
  wires:
  I*w/1 -> Reshape5/1
  I/1 -> I*w/1, Product2/2
  Reshape4/1 -> I*w/2
  I_dot/1 -> Idot*w/1
  Idot*w/1 -> Reshape3/1
  Reshape2/1 -> Idot*w/2
  Reshape/1 -> pdot qdot rdot/1
  p q r/1 -> CrossProduct3/1, Reshape4/1, Reshape2/1
  Product2/1 -> Reshape/1
  Sum2/1 -> Reshape1/1
  Moments/1 -> Sum2/1
  Reshape3/1 -> Sum2/2
  CrossProduct3/1 -> Sum2/3
  Reshape5/1 -> CrossProduct3/2
  Reshape1/1 -> Product2/1

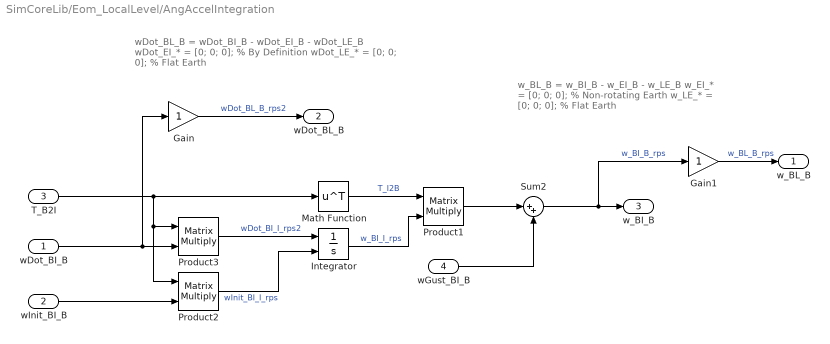
== system SimCoreLib/Eom_LocalLevel/AngAccelIntegration ==
  note: w_BL_B = w_BI_B - w_EI_B - w_LE_B
      | w_EI_* = [0; 0; 0]; % Non-rotating Earth
      | w_LE_* = [0; 0; 0]; % Flat Earth
  note: wDot_BL_B = wDot_BI_B - wDot_EI_B - wDot_LE_B
      | wDot_EI_* = [0; 0; 0]; % By Definition
      | wDot_LE_* = [0; 0; 0]; % Flat Earth
  wDot_BI_B : Inport
  wInit_BI_B : Inport  Port=2
  T_B2I : Inport  Port=3
  wGust_BI_B : Inport  Port=4
  Gain : Gain
  Gain1 : Gain
  Integrator : Integrator  InitialConditionSource=external  ContinuousStateAttributes='wState_BI_I_rps'
      settings: AttributesFormatString=State: %<ContinuousStateAttributes>
  Math Function : Math  Operator=transpose  SaturateOnIntegerOverflow=on
  Product1 : Product  Inputs=**  Multiplication=Matrix(*)  RndMeth=Zero
  Product2 : Product  Inputs=**  Multiplication=Matrix(*)  RndMeth=Zero
  Product3 : Product  Inputs=**  Multiplication=Matrix(*)  RndMeth=Zero
  Sum2 : Sum  Inputs=|++  SaturateOnIntegerOverflow=on
  w_BL_B : Outport
  wDot_BL_B : Outport  Port=2
  w_BI_B : Outport  Port=3
  wires:
  Product1/1 -> Sum2/1
  wGust_BI_B/1 -> Sum2/2
  Gain/1 -> wDot_BL_B/1  "wDot_BL_B_rps2"
  Gain1/1 -> w_BL_B/1  "w_BL_B_rps"
  wDot_BI_B/1 -> Product3/2, Gain/1
  Product2/1 -> Integrator/2  "wInit_BI_I_rps"
  wInit_BI_B/1 -> Product2/2
  Integrator/1 -> Product1/2  "w_BI_I_rps"
  T_B2I/1 -> Math Function/1, Product3/1, Product2/1
  Product3/1 -> Integrator/1  "wDot_BI_I_rps2"
  Math Function/1 -> Product1/1  "T_I2B"
  Sum2/1 -> w_BI_B/1, Gain1/1  "w_BI_B_rps"

== system SimCoreLib/Eom_LocalLevel/AngVelIntegration_Quat ==
  w_BL_B : Inport
  sInit_BL : Inport  Port=2
  Euler2Quat : OpenFlightUtilLib/Transformations/Euler2Quat
  NormL2 : OpenFlightUtilLib/Math/NormL2
  Product2 : Product  Inputs=*/  RndMeth=Zero
  Quat2DCM321 : OpenFlightUtilLib/Transformations/Quat2DCM
  Quat2Euler : OpenFlightUtilLib/Transformations/Quat2Euler
  QuatDeriv : OpenFlightUtilLib/Transformations/QuatDeriv
  QuatInt : OpenFlightUtilLib/Transformations/QuatInt
  T_L2B : Outport
  s_BL : Outport  Port=2
  wires:
  sInit_BL/1 -> Euler2Quat/1
  Quat2Euler/1 -> s_BL/1  "s_BL_rad"
  Quat2DCM321/1 -> T_L2B/1  "T_L2B"
  NormL2/1 -> Product2/2
  QuatDeriv/1 -> QuatInt/1  "quatDot_BL_nd"
  QuatInt/1 -> Product2/1, NormL2/1
  Product2/1 -> Quat2Euler/1, Quat2DCM321/1, QuatDeriv/1  "quat_BL_nd"
  Euler2Quat/1 -> QuatInt/2  "quatInit_BL_nd"
  w_BL_B/1 -> QuatDeriv/2

== system SimCoreLib/Eom_LocalLevel/Force2Accel ==
  w_BI_B : Inport
  fExt : Inport  Port=2
  m : Inport  Port=3
  mDot : Inport  Port=4
  aGrav_BI_B : Inport  Port=5
  v_BI_B : Inport  Port=6
  Sum2 : Sum  Inputs=|++  SaturateOnIntegerOverflow=on
  TransMomentumInv : OpenFlightUtilLib/Kinematics and Dynamics/TransMomentumInv
  aExt_BI_B : Outport
  a_BI_B : Outport  Port=2
  wires:
  fExt/1 -> TransMomentumInv/3
  v_BI_B/1 -> TransMomentumInv/1
  TransMomentumInv/1 -> Sum2/1, aExt_BI_B/1  "aExt_BI_B_mps2"
  w_BI_B/1 -> TransMomentumInv/5
  mDot/1 -> TransMomentumInv/4
  m/1 -> TransMomentumInv/2
  aGrav_BI_B/1 -> Sum2/2
  Sum2/1 -> a_BI_B/1  "a_BI_B_mps2"

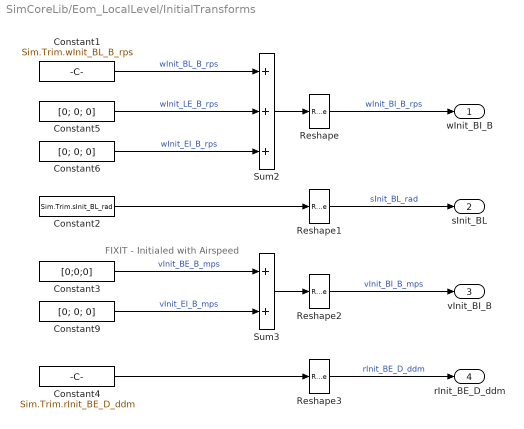
== system SimCoreLib/Eom_LocalLevel/InitialTransforms ==
  note: FIXIT - Initialed with Airspeed
  Constant1 : Constant  Value=Sim.Trim.wInit_BL_B_rps
      settings: AttributesFormatString=%<Value>
  Constant2 : Constant  Value=Sim.Trim.sInit_BL_rad
      settings: AttributesFormatString=%<Value>
  Constant3 : Constant  Value=[0;0;0]
      settings: AttributesFormatString=%<Value>
  Constant4 : Constant  Value=Sim.Trim.rInit_BE_D_ddm
      settings: AttributesFormatString=%<Value>
  Constant5 : Constant  Value=[0; 0; 0]
      settings: AttributesFormatString=%<Value>
  Constant6 : Constant  Value=[0; 0; 0]
      settings: AttributesFormatString=%<Value>
  Constant9 : Constant  Value=[0; 0; 0]
      settings: AttributesFormatString=%<Value>
  Reshape{,1..3} (4 alike) : Reshape  OutputDimensionality=Column vector (2-D)  OutputDimensions=[3,1]
  Sum2 : Sum  Inputs=+++  SaturateOnIntegerOverflow=on
  Sum3 : Sum  SaturateOnIntegerOverflow=on
  wInit_BI_B : Outport
  sInit_BL : Outport  Port=2
  vInit_BI_B : Outport  Port=3
  rInit_BE_D_ddm : Outport  Port=4
  wires:
  Reshape3/1 -> rInit_BE_D_ddm/1  "rInit_BE_D_ddm"
  Reshape2/1 -> vInit_BI_B/1  "vInit_BI_B_mps"
  Reshape1/1 -> sInit_BL/1  "sInit_BL_rad"
  Sum2/1 -> Reshape/1
  Sum3/1 -> Reshape2/1
  Constant9/1 -> Sum3/2  "vInit_EI_B_mps"
  Constant6/1 -> Sum2/3  "wInit_EI_B_rps"
  Constant5/1 -> Sum2/2  "wInit_LE_B_rps"
  Reshape/1 -> wInit_BI_B/1  "wInit_BI_B_rps"
  Constant4/1 -> Reshape3/1
  Constant3/1 -> Sum3/1  "vInit_BE_B_mps"
  Constant2/1 -> Reshape1/1
  Constant1/1 -> Sum2/1  "wInit_BL_B_rps"

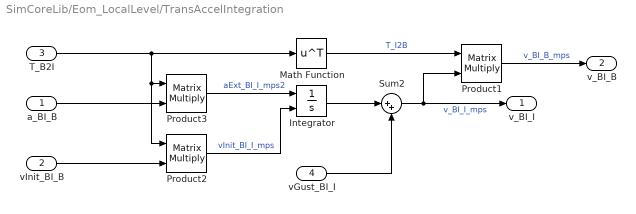
== system SimCoreLib/Eom_LocalLevel/TransAccelIntegration ==
  a_BI_B : Inport
  vInit_BI_B : Inport  Port=2
  T_B2I : Inport  Port=3
  vGust_BI_I : Inport  Port=4
  Integrator : Integrator  InitialConditionSource=external  ContinuousStateAttributes='vState_BI_I_mps'
      settings: AttributesFormatString=State: %<ContinuousStateAttributes>
  Math Function : Math  Operator=transpose  SaturateOnIntegerOverflow=on
  Product1 : Product  Inputs=**  Multiplication=Matrix(*)  RndMeth=Zero
  Product2 : Product  Inputs=**  Multiplication=Matrix(*)  RndMeth=Zero
  Product3 : Product  Inputs=**  Multiplication=Matrix(*)  RndMeth=Zero
  Sum2 : Sum  Inputs=|++  SaturateOnIntegerOverflow=on
  v_BI_I : Outport
  v_BI_B : Outport  Port=2
  wires:
  Integrator/1 -> Sum2/1
  vGust_BI_I/1 -> Sum2/2
  Sum2/1 -> v_BI_I/1, Product1/2  "v_BI_I_mps"
  vInit_BI_B/1 -> Product2/2
  a_BI_B/1 -> Product3/2
  T_B2I/1 -> Product3/1, Product2/1, Math Function/1
  Math Function/1 -> Product1/1  "T_I2B"
  Product1/1 -> v_BI_B/1  "v_BI_B_mps"
  Product3/1 -> Integrator/1  "aExt_BI_I_mps2"
  Product2/1 -> Integrator/2  "vInit_BI_I_mps"

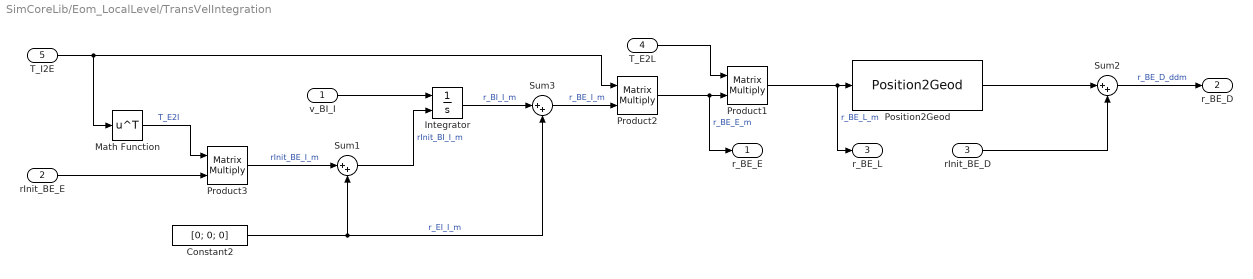
== system SimCoreLib/Eom_LocalLevel/TransVelIntegration ==
  v_BI_I : Inport
  rInit_BE_E : Inport  Port=2
  rInit_BE_D : Inport  Port=3
  T_E2L : Inport  Port=4
  T_I2E : Inport  Port=5
  Constant2 : Constant  Value=[0; 0; 0]
      settings: AttributesFormatString=%<Value>
  Integrator : Integrator  InitialConditionSource=external  ContinuousStateAttributes='rInit_BI_I_m'
      settings: AttributesFormatString=State: %<ContinuousStateAttributes>
  Math Function : Math  Operator=transpose  SaturateOnIntegerOverflow=on
  Position2Geod : SimCoreLib/Position2Geod
  Product1 : Product  Inputs=**  Multiplication=Matrix(*)  RndMeth=Zero
  Product2 : Product  Inputs=**  Multiplication=Matrix(*)  RndMeth=Zero
  Product3 : Product  Inputs=**  Multiplication=Matrix(*)  RndMeth=Zero
  Sum1 : Sum  Inputs=|++
  Sum2 : Sum  Inputs=|++
  Sum3 : Sum  Inputs=|++
  r_BE_E : Outport
  r_BE_D : Outport  Port=2
  r_BE_L : Outport  Port=3
  wires:
  Sum1/1 -> Integrator/2  "rInit_BI_I_m"
  Product3/1 -> Sum1/1  "rInit_BE_I_m"
  Math Function/1 -> Product3/1  "T_E2I"
  T_I2E/1 -> Product2/1, Math Function/1
  Product2/1 -> Product1/2, r_BE_E/1  "r_BE_E_m"
  Constant2/1 -> Sum3/2, Sum1/2  "r_EI_I_m"
  Sum3/1 -> Product2/2  "r_BE_I_m"
  rInit_BE_E/1 -> Product3/2
  rInit_BE_D/1 -> Sum2/2
  Sum2/1 -> r_BE_D/1  "r_BE_D_ddm"
  Product1/1 -> r_BE_L/1, Position2Geod/1  "r_BE_L_m"
  T_E2L/1 -> Product1/1
  Position2Geod/1 -> Sum2/1
  Integrator/1 -> Sum3/1  "r_BI_I_m"
  v_BI_I/1 -> Integrator/1

== system SimCoreLib/FlowConditions/ApplyWind ==
  note: aWind_BA_B = a_BI_B - a_EI_B - T_L2B * a_AE_L;
      |
      | a_EI_B = [0; 0; 0];
      | a_AE_L = aWind = 0; % Steady Wind
  note: vWind_BA_B = v_BE_B - T_L2B * v_AE_L;
      |
      | v_AE_L = vWind;
  Eom : Inport
  Env : Inport  Port=2
  Bus Selector1 : BusSelector  OutputSignals=v_BE_B_mps,T_L2B
  Bus Selector2 : BusSelector  OutputSignals=a_BI_B_mps2
  Bus Selector4 : BusSelector  OutputSignals=BusAtmos.vWind_mps
  Gain : Gain
  Product1 : Product  Inputs=**  Multiplication=Matrix(*)  RndMeth=Zero
  Sum1 : Sum  Inputs=|+-  SaturateOnIntegerOverflow=on
  v_BA_B : Outport
  a_BA_B : Outport  Port=2
  wires:
  Gain/1 -> a_BA_B/1  "a_BA_B_mps2"
  Bus Selector2/1 -> Gain/1  "<a_BI_B_mps2>"
  Sum1/1 -> v_BA_B/1  "v_BA_B_mps"
  Product1/1 -> Sum1/2  "v_AI_B_mps"
  Bus Selector1/2 -> Product1/1  "<T_L2B>"
  Bus Selector4/1 -> Product1/2  "<vWind_mps>"
  Bus Selector1/1 -> Sum1/1  "<v_BE_B_mps>"
  Eom/1 -> Bus Selector1/1, Bus Selector2/1
  Env/1 -> Bus Selector4/1

== system SimCoreLib/Nav_Simple/GeoidModel_EGM96 ==
  r_BI_D : Inport
  Demux2 : Demux  Outputs=3
  Look-Up Table (2-D) : Lookup2D  RowIndex=Lat  ColumnIndex=Lon  Table=Alterr'  SaturateOnIntegerOverflow=on  InputSameDT=on
  Sum : Sum  Inputs=|+++
  WGS-84 correction : Constant  Value=-0.53
  Alt MSL : Outport
  wires:
  WGS-84 correction/1 -> Sum/3
  Look-Up Table (2-D)/1 -> Sum/1
  Sum/1 -> Alt MSL/1
  Demux2/3 -> Sum/2
  r_BI_D/1 -> Demux2/1
  Demux2/1 -> Look-Up Table (2-D)/1
  Demux2/2 -> Look-Up Table (2-D)/2

== system SimCoreLib/Nav_Simple/Terrain ==
  Alt : Inport
  Alt Grnd : Inport  Port=2
  Sum : Sum  Inputs=|+-  SaturateOnIntegerOverflow=on  InputSameDT=on  OutDataTypeStr=Inherit: Same as first input
  Alt AGL : Outport
  wires:
  Alt/1 -> Sum/1
  Sum/1 -> Alt AGL/1  "altAgl_m"
  Alt Grnd/1 -> Sum/2

== system SimCoreLib/Eom_AeroBlock/Euler Angle Bounds/2pi Bound ==
  In : Inport
  2pi : Constant  Value=2*pi
  Math Function2 : Math  Operator=mod  SaturateOnIntegerOverflow=on
  Out : Outport
  wires:
  Math Function2/1 -> Out/1
  2pi/1 -> Math Function2/2
  In/1 -> Math Function2/1

== system SimCoreLib/Eom_AeroBlock/Euler Angle Bounds/pi Bound ==
  In : Inport
  Math Function1 : Math  Operator=mod  SaturateOnIntegerOverflow=on
  Sum3 : Sum  Inputs=|+-  SaturateOnIntegerOverflow=on  InputSameDT=on  OutDataTypeStr=Inherit: Same as first input
  Sum4 : Sum  Inputs=|++  SaturateOnIntegerOverflow=on  InputSameDT=on  OutDataTypeStr=Inherit: Same as first input
  pi2 : Constant  Value=pi
  pi3 : Constant  Value=2*pi
  Out : Outport
  wires:
  Math Function1/1 -> Sum3/1
  pi3/1 -> Math Function1/2
  In/1 -> Sum4/1
  Sum4/1 -> Math Function1/1
  pi2/1 -> Sum4/2, Sum3/2
  Sum3/1 -> Out/1

== system SimCoreLib/Eom_AeroBlock/Euler Angle Bounds/pi//2 Bound ==
  In : Inport
  Math Function : Math  Operator=mod  SaturateOnIntegerOverflow=on
  Sum1 : Sum  Inputs=|+-  SaturateOnIntegerOverflow=on  InputSameDT=on  OutDataTypeStr=Inherit: Same as first input
  Sum2 : Sum  Inputs=|++  SaturateOnIntegerOverflow=on  InputSameDT=on  OutDataTypeStr=Inherit: Same as first input
  pi : Constant  Value=pi/2
  pi1 : Constant  Value=pi
  Out : Outport
  wires:
  Sum1/1 -> Out/1
  pi/1 -> Sum1/2, Sum2/2
  Sum2/1 -> Math Function/1
  In/1 -> Sum2/1
  pi1/1 -> Math Function/2
  Math Function/1 -> Sum1/1

== system SimCoreLib/Eom_Copy/Euler Angle Bounds/2pi Bound ==
  In : Inport
  2pi : Constant  Value=2*pi
  Math Function2 : Math  Operator=mod  SaturateOnIntegerOverflow=on
  Out : Outport
  wires:
  In/1 -> Math Function2/1
  2pi/1 -> Math Function2/2
  Math Function2/1 -> Out/1

== system SimCoreLib/Eom_Copy/Euler Angle Bounds/pi Bound ==
  In : Inport
  Math Function1 : Math  Operator=mod  SaturateOnIntegerOverflow=on
  Sum3 : Sum  Inputs=|+-  SaturateOnIntegerOverflow=on  InputSameDT=on  OutDataTypeStr=Inherit: Same as first input
  Sum4 : Sum  Inputs=|++  SaturateOnIntegerOverflow=on  InputSameDT=on  OutDataTypeStr=Inherit: Same as first input
  pi2 : Constant  Value=pi
  pi3 : Constant  Value=2*pi
  Out : Outport
  wires:
  Sum3/1 -> Out/1
  pi2/1 -> Sum3/2, Sum4/2
  Sum4/1 -> Math Function1/1
  In/1 -> Sum4/1
  pi3/1 -> Math Function1/2
  Math Function1/1 -> Sum3/1

== system SimCoreLib/Eom_Copy/Euler Angle Bounds/pi//2 Bound ==
  In : Inport
  Math Function : Math  Operator=mod  SaturateOnIntegerOverflow=on
  Sum1 : Sum  Inputs=|+-  SaturateOnIntegerOverflow=on  InputSameDT=on  OutDataTypeStr=Inherit: Same as first input
  Sum2 : Sum  Inputs=|++  SaturateOnIntegerOverflow=on  InputSameDT=on  OutDataTypeStr=Inherit: Same as first input
  pi : Constant  Value=pi/2
  pi1 : Constant  Value=pi
  Out : Outport
  wires:
  Math Function/1 -> Sum1/1
  pi1/1 -> Math Function/2
  In/1 -> Sum2/1
  Sum2/1 -> Math Function/1
  pi/1 -> Sum2/2, Sum1/2
  Sum1/1 -> Out/1

== system SimCoreLib/Eom_Copy/Euler and DCM/phidot thetadot psidot ==
  phi theta psi : Inport
  p q r : Inport  Port=2
  Mux1 : Mux  Inputs=[3 3]
  Mux4 : Mux  Inputs=3
  phi dot : Fcn  Expr=u(1)+(u(2)*sin(u(4))+u(3)*cos(u(4)))*tan(u(5))
  psi dot : Fcn  Expr=(u(2)*sin(u(4))+u(3)*cos(u(4)))/cos(u(5))
  theta dot : Fcn  Expr=u(2)*cos(u(4))-u(3)*sin(u(4))
  phidt thetadt psidt : Outport  InitialOutput=0
  wires:
  p q r/1 -> Mux1/1
  psi dot/1 -> Mux4/3
  theta dot/1 -> Mux4/2
  phi dot/1 -> Mux4/1
  Mux1/1 -> phi dot/1, theta dot/1, psi dot/1
  Mux4/1 -> phidt thetadt psidt/1
  phi theta psi/1 -> Mux1/2
